simulink model "dds_cwg_bu"  (R2016b)
(part 2 of 89)

  control/10(in_adc_snap_trig_select) -> pipeline39/1(d)
  pipeline39/1(q) -> [adc_snap_trig_source]
  pipeline59/1(q) -> [ct_tvg_en]
  control/11(in_ct_tvg_en) -> pipeline59/1(d)
  pipeline52/1(q) -> [up_dbg_rst]
  control/12(in_unpack_debug_reset) -> pipeline52/1(d)
  control/13(in_cd_bypass) -> pipeline131/1(d)
  pipeline131/1(q) -> [cd_bypass]
  pipeline93/1(q) -> [tvg_adc1_en]
  control/6(in_tvg_adc1) -> pipeline93/1(d)
  control/14(in_gbe_stopmux) -> pipeline27/1(d)
  pipeline27/1(q) -> [gbe_stopmux]
  control/15(in_pfb_bypass) -> pipeline66/1(d)
  pipeline66/1(q) -> [pfb_bypass]
  control/16(in_ts_tvg_en) -> pipeline148/1(d)
  pipeline148/1(q) -> [ts_tvg_en]
  control/17(in_force_gbe_txen) -> pipeline21/1(d)
  pipeline21/1(q) -> [force_gbe_txen]
  control/18(in_snap_stop_mux_sel) -> pipeline127/1(d)
  control/19(in_snap_reord_mux_we_sel) -> pipeline128/1(d)
  pipeline127/1(q) -> [snap_stop_mux_sel]
  pipeline128/1(q) -> [snap_reord_mux_we_sel]
  control/20(in_local_time_source) -> pipeline16/1(d)
  edge_detect8/1(out) -> pipeline164/1(d)
  pipeline164/1(q) -> [local_time_capture]
  pipeline16/1(q) -> [local_time_src]
  control/21(in_local_time_capture) -> edge_detect8/1(in)
  control/22(in_time_diff_check_en) -> pipeline47/1(d)
  pipeline47/1(q) -> [time_diff_check_en]
  control/23(in_auto_rst_enable) -> pipeline132/1(d)
  pipeline132/1(q) -> [auto_rst_enable]
  pipeline155/1(q) -> [pipeline_stall]
  control/24(in_pipeline_stall) -> pipeline155/1(d)
  [board_in_fault] -> Inverter/1
  Inverter/1 -> Logical7/1
  Constant18/1 -> [board_in_fault]
  Constant22/1 -> [s256_d]
  Constant23/1 -> [s256_v]
  Constant24/1 -> [s256_eof]
  Constant25/1 -> [s256_port]
  Constant26/1 -> [s256_ip]
  Constant27/1 -> fft_fwd_inv/1(sim_1)
  nb_pfb/5(new_spec) -> Goto5/1
  Relational2/1 -> [osc_temp_dv]
  fft_shift/1(in_fft_shift) -> pipeline15/1(d)
  pipeline15/1(q) -> [fft_shift]
  Constant28/1 -> fft_shift/1(sim_1)
  From26/1 -> nb_pfb/5(fft_shift)
  Gateway Out24/1 -> To Workspace25/1
  bus_expand3/1(msb_out8) -> Gateway Out24/1
  Gateway Out10/1 -> To Workspace10/1
  bus_expand3/2(out7) -> Gateway Out10/1
  Gateway Out25/1 -> To Workspace24/1
  bus_expand3/3(out6) -> Gateway Out25/1
  Gateway Out26/1 -> To Workspace26/1
  bus_expand3/4(out5) -> Gateway Out26/1
  Gateway Out27/1 -> To Workspace27/1
  bus_expand3/5(out4) -> Gateway Out27/1
  Gateway Out28/1 -> To Workspace28/1
  bus_expand3/6(out3) -> Gateway Out28/1
  Gateway Out29/1 -> To Workspace29/1
  bus_expand3/7(out2) -> Gateway Out29/1
  Gateway Out30/1 -> To Workspace30/1
  bus_expand3/8(lsb_out1) -> Gateway Out30/1
  cwg3/1(bus_out) -> [dds80], bus_expand3/1(bus_in)
  Constant2/1 -> freq_cwg_osc1/1(sim_1)
  Constant30/1 -> freq_cwg_osc/1(sim_1)
  Gateway Out32/1 -> To Workspace33/1
  bus_expand4/1(msb_out8) -> Gateway Out32/1
  Gateway Out31/1 -> To Workspace31/1
  bus_expand4/2(out7) -> Gateway Out31/1
  Gateway Out33/1 -> To Workspace32/1
  bus_expand4/3(out6) -> Gateway Out33/1
  Gateway Out34/1 -> To Workspace34/1
  bus_expand4/4(out5) -> Gateway Out34/1
  Gateway Out37/1 -> To Workspace37/1
  bus_expand4/5(out4) -> Gateway Out37/1
  Gateway Out38/1 -> To Workspace38/1
  bus_expand4/6(out3) -> Gateway Out38/1
  Gateway Out39/1 -> To Workspace39/1
  bus_expand4/7(out2) -> Gateway Out39/1
  Gateway Out40/1 -> To Workspace40/1
  bus_expand4/8(lsb_out1) -> Gateway Out40/1
  cwg4/1(bus_out) -> bus_expand4/1(bus_in)
  freq_cwg_osc3/1(in_frequency) -> cwg4/1(freq)
  Constant31/1 -> freq_cwg_osc3/1(sim_1)
  [fft_shift] -> nb_pfb1/5(fft_shift)
  [ddc_dvalid] -> nb_pfb1/4(dvalid)
  [ddc_pol1] -> nb_pfb1/3(pol1)
  [ddc_pol0] -> nb_pfb1/2(pol0)
  [ddc_sync] -> nb_pfb1/1(sync)
  edge_detect3/1(out) -> Register1/3, Register1/1
  Delay7/1 -> edge_detect3/1(in)
  [dds80] -> DDC/4(osc0), DDC/7(osc1)
  [ddc_dv_in] -> DDC/2(dvalid)
  [ddc_sync_in] -> DDC/1(sync), Gateway Out74/1
  [cwg80] -> DDC/6(pol1_data), DDC/3(pol0_data)
  Constant32/1 -> freq_cwg_osc2/1(sim_1)
  freq_cwg_osc2/1(in_frequency) -> pipeline19/1(d)
  pipeline19/1(q) -> cwg3/1(freq)
